simulink model "cartpole_lqg_blockdiagram"  (R2026a)
settings: Solver=VariableStepAuto
values from neighbouring files (symbols this model uses):
  A = [0 1 0 0 ... (first row only)    [cartpole_lqg_Kmatrix.m]
  B = [0; 1/M; 0; -1/(L*M)]    [cartpole_lqg_Kmatrix.m]
  C = eye(4)    [cartpole_lqg_Kmatrix.m]
  D = zeros(4, 1)    [cartpole_lqg_Kmatrix.m]
  K = lqr(A, B, Q, R)    [cartpole_lqg_Kmatrix.m]
  R_kalman = diag([0.001, 0.001, 0.001, 0.001])    [cartpole_lqg_Kmatrix.m]
undefined symbols (not defined in the file or in its folder): Discrete, Time
libraries: simulink x2, ctrlSharedLib x1
settings Model: Creator=billy  LastModifiedBy=billy

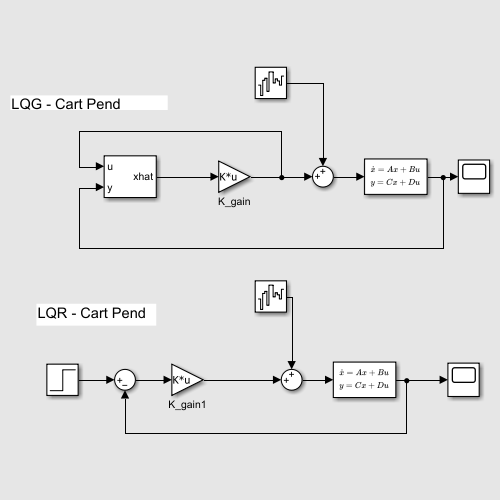
[thumbnail: Simulink's stored preview of the top-level diagram]
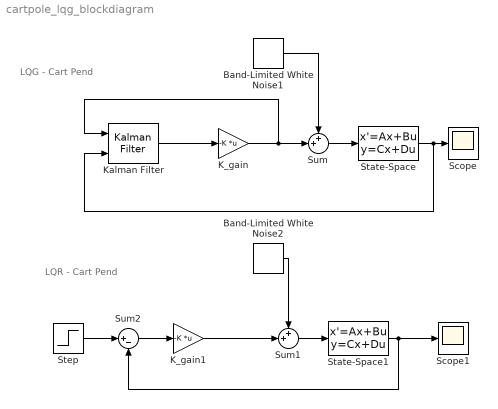
== system cartpole_lqg_blockdiagram ==
  note: LQR - Cart Pend
  note: LQG - Cart Pend
  Band-Limited White Noise1 : simulink/Sources/Band-Limited White Noise  Cov=[0.1]  Ts=0.1  seed=[23341]
  Band-Limited White Noise2 : simulink/Sources/Band-Limited White Noise  Cov=[0.1]  Ts=0.1  seed=[23341]
  K_gain : Gain  Gain=-K  Multiplication=Matrix(K*u)
  K_gain1 : Gain  Gain=-K  Multiplication=Matrix(K*u)
  Kalman Filter : ctrlSharedLib/Kalman Filter  TimeDomain=Discrete-Time  UseCurrentEstimator=on  ModelSource=Individual A, B, C, D matrices  ModelSourceVariable=ss(0.95,1,1,0,1)  A=A  B=B  C=C  D=D  NumberOfStates=1  NumberOfInputs=1  NumberOfOutputs=1  Ts=-1  InitialEstimateSource=Dialog  X0=0  P0=10  UseK=off  UseGH=off  G=1  TimeInvariantG=on  H=0  TimeInvariantH=on  NumberOfProcessNoiseInputs=1  Q=Q_kalman  TimeInvariantQ=on  R=R_kalman  TimeInvariantR=on  N=0  TimeInvariantN=on  AddInputPort=on  AddEnablePort=off  OutputEstimatedY=off  OutputP=off
  Scope : Scope
      settings: ActiveDisplayYMinimum=-4.7359194339347333E+6  ActiveDisplayYMaximum=4.860728366681356E+6
  Scope1 : Scope
      settings: ActiveDisplayYMinimum=-4.7359194339347333E+6  ActiveDisplayYMaximum=4.860728366681356E+6
  State-Space : StateSpace  A=A  B=B  C=C  D=D  InitialCondition=0
  State-Space1 : StateSpace  A=A  B=B  C=C  D=D  InitialCondition=0
  Step : Step  SampleTime=0
  Sum : Sum  Inputs=++|
  Sum1 : Sum  Inputs=++|
  Sum2 : Sum  Inputs=|+-
  wires:
  K_gain/1 -> Sum/2, Kalman Filter/1
  Kalman Filter/1 -> K_gain/1
  Sum/1 -> State-Space/1
  Band-Limited White Noise1/1 -> Sum/1
  State-Space/1 -> Scope/1, Kalman Filter/2
  State-Space1/1 -> Sum2/2, Scope1/1
  Sum1/1 -> State-Space1/1
  K_gain1/1 -> Sum1/2
  Sum2/1 -> K_gain1/1
  Step/1 -> Sum2/1
  Band-Limited White Noise2/1 -> Sum1/1
